simulink model "example_of_data_type_conversion"  (R2021a)
settings: Solver=VariableStepAuto  StartTime=0.0  StopTime=10.0  RelTol=1e-3
settings Model: Creator=YasserNet  LastModifiedBy=YasserNet

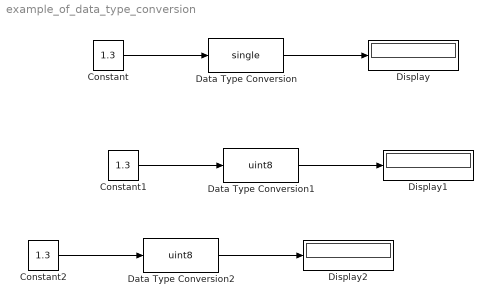
== system example_of_data_type_conversion ==
  Constant : Constant  Value=1.3  OutDataTypeStr=double
  Constant1 : Constant  Value=1.3  OutDataTypeStr=double
  Constant2 : Constant  Value=1.3  OutDataTypeStr=uint16
  Data Type Conversion : DataTypeConversion  OutDataTypeStr=single
  Data Type Conversion1 : DataTypeConversion  OutDataTypeStr=uint8  RndMeth=Round
  Data Type Conversion2 : DataTypeConversion  OutDataTypeStr=uint8  RndMeth=Round
  Display : Display
  Display1 : Display
  Display2 : Display
  wires:
  Data Type Conversion/1 -> Display/1
  Constant/1 -> Data Type Conversion/1
  Data Type Conversion1/1 -> Display1/1
  Constant1/1 -> Data Type Conversion1/1
  Constant2/1 -> Data Type Conversion2/1
  Data Type Conversion2/1 -> Display2/1
